simulink model "Filter"  (R2023b)
settings: Solver=ode45  StartTime=0.0  StopTime=10.0  RelTol=1e-3  EnableMultiTasking=on
libraries: dspfdesign x2
settings Model: Creator=Karan  LastModifiedBy=Crystal Shop
settings SolverCC: AlgebraicLoopSolver=TrustRegion
settings DataIOCC: LimitDataPoints=on  SaveFormat=Array  ReturnWorkspaceOutputs=off
settings OptimizationCC: LifeSpan=inf
settings DebuggingCC: SolverPrmCheckMsg=warning  UnconnectedInputMsg=warning  UnconnectedOutputMsg=warning  UnconnectedLineMsg=warning  SFUnexpectedBacktrackingDiag=warning  SFNoUnconditionalDefaultTransitionDiag=warning  SFExecutionAtInitializationDiag=none  ArithmeticOperatorsInVariantConditions=warning
settings HardwareCC: ProdBitPerPointer=32  ProdBitPerSizeT=32  ProdBitPerPtrDiffT=32  ProdLargestAtomicFloat=None  ProdIntDivRoundTo=Undefined  ProdEndianess=Unspecified  ProdWordSize=32  ProdHWDeviceType=32-bit Generic
settings ModelReferenceCC: PropagateSignalLabelsOutOfModel=off
settings SFSimCC: SimUseLocalCustomCode=off  CustomCodeUndefinedFunction=UseInterfaceOnly
settings RTWCC: RTWUseLocalCustomCode=off
settings CodeAppCC: StateflowObjectComments=on
settings GRTTargetCC: TargetLangStandard=C89/C90 (ANSI)
settings ConfigComp: CovMetricSettings=dw  CovSaveCumulativeToWorkspaceVar=on  CovSaveSingleToWorkspaceVar=on  CovExternalEMLEnable=off  CovSFcnEnable=off

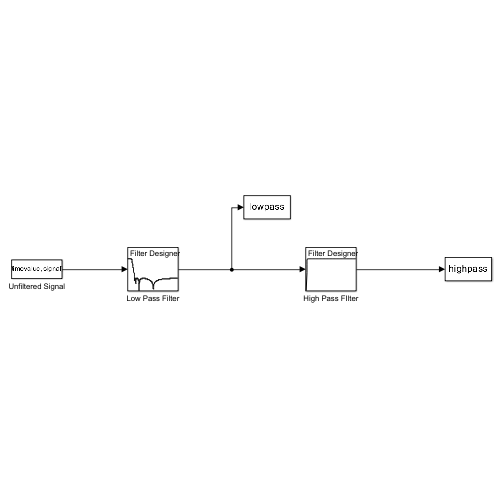
[thumbnail: Simulink's stored preview of the top-level diagram]
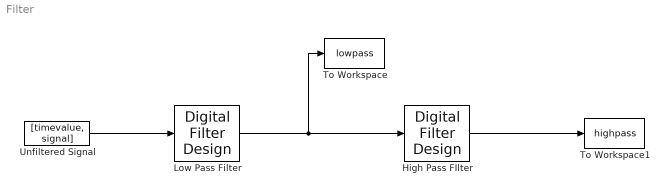
== system Filter ==
  High Pass FIlter : dspfdesign/Digital Filter Design  mwdsp_browser_bugfix_var=off
  Low Pass Filter : dspfdesign/Digital Filter Design  mwdsp_browser_bugfix_var=off
  To Workspace : ToWorkspace  VariableName=lowpass  SampleTime=1/800
      settings: Save2DSignal=2-D array (concatenate along first dimension)
  To Workspace1 : ToWorkspace  VariableName=highpass  SampleTime=1/800
      settings: Save2DSignal=2-D array (concatenate along first dimension)
  Unfiltered Signal : FromWorkspace  VariableName=[timevalue, signal]  SampleTime=1/800
  wires:
  Unfiltered Signal/1 -> Low Pass Filter/1
  Low Pass Filter/1 -> High Pass FIlter/1, To Workspace/1
  High Pass FIlter/1 -> To Workspace1/1
